simulink model "problem2"  (R2025b)
settings: Solver=VariableStepAuto  StartTime=0.0  StopTime=100.0  RelTol=1e-3
settings Model: Creator=Maria Islam  LastModifiedBy=Maria Islam

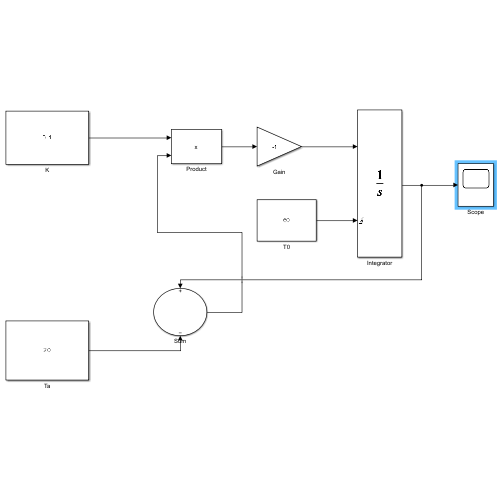
[thumbnail: Simulink's stored preview of the top-level diagram]
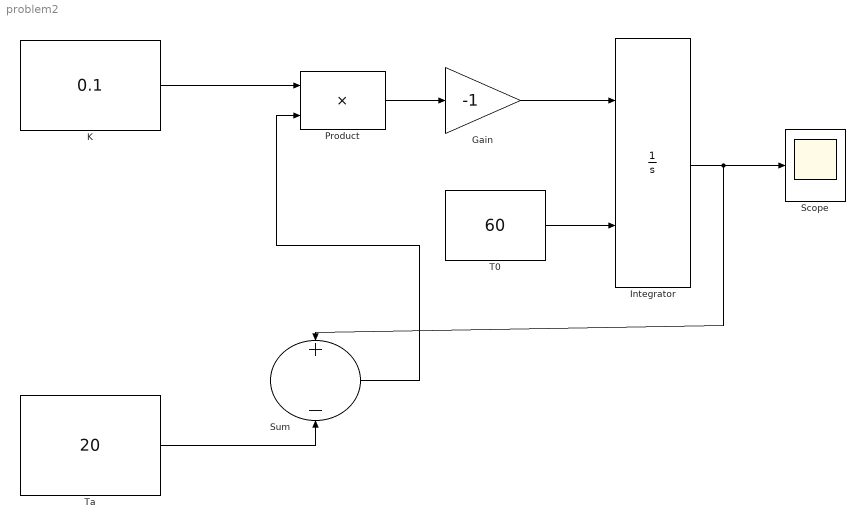
== system problem2 ==
  Gain : Gain  Gain=-1
  Integrator : Integrator  ExternalReset=rising  InitialCondition=60
  K : Constant  Value=0.1
  Product : Product
  Scope : Scope
      settings: ActiveDisplayYMinimum=18.494808566596344  ActiveDisplayYMaximum=90.592441602111734
  Sum : Sum  Inputs=+-
  T0 : Constant  Value=60
  Ta : Constant  Value=20
  wires:
  Ta/1 -> Sum/2
  K/1 -> Product/1
  Sum/1 -> Product/2
  Product/1 -> Gain/1
  Gain/1 -> Integrator/1
  T0/1 -> Integrator/2
  Integrator/1 -> Sum/1, Scope/1
